simulink model "adaptive_feedforward"  (R2025b)
settings: Solver=FixedStepAuto  StartTime=0.0  StopTime=20  FixedStep=Ts  RelTol=1e-3
InitFcn:
  | design_adaptive_ff
values from neighbouring files (symbols this model uses):
  gamma = 1    [design_adaptive_ff.m]
  gamma_0 = 1    [design_adaptive_ff.m]
settings Model: Creator=10120  LastModifiedBy=10120

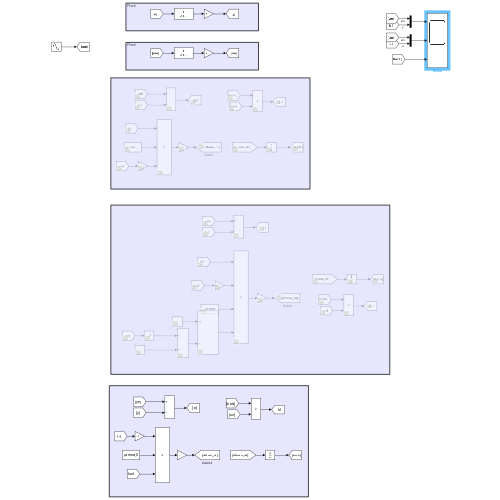
[thumbnail: Simulink's stored preview of the top-level diagram]
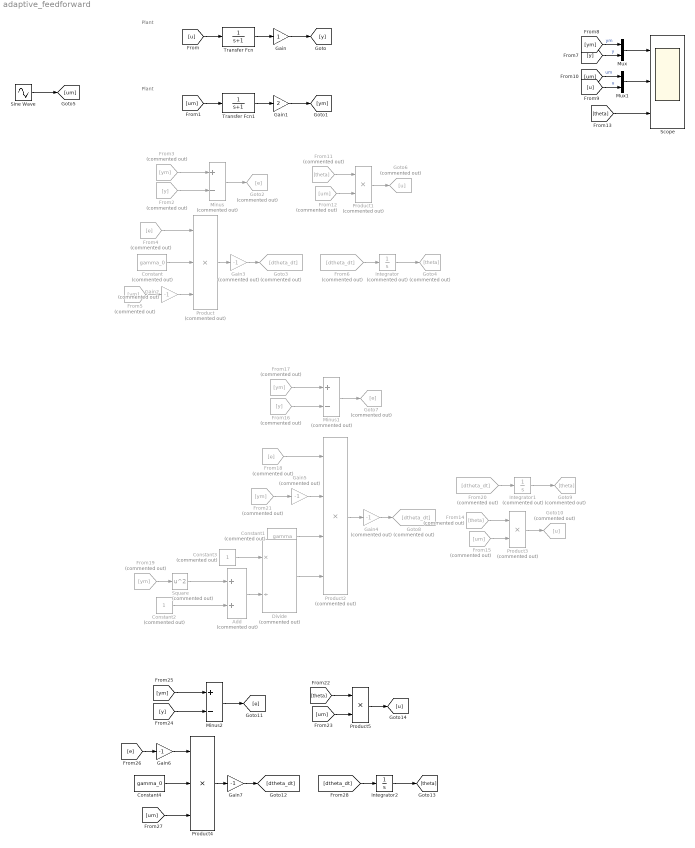
== system adaptive_feedforward ==
  note: Plant
  note: Plant
  Add : Sum  Commented=on
  Constant : Constant  Commented=on  Value=gamma_0
  Constant1 : Constant  Commented=on  Value=gamma
  Constant2 : Constant  Commented=on
  Constant3 : Constant  Commented=on
  Constant4 : Constant  Value=gamma_0
  Divide : Product  Commented=on  Inputs=*/
  From11 : From  Commented=on  GotoTag=theta
  From12 : From  Commented=on  GotoTag=um
  From14 : From  Commented=on  GotoTag=theta
  From15 : From  Commented=on  GotoTag=um
  From16 : From  Commented=on  GotoTag=y
  From{3,5,17,19,21} (5 alike) : From  Commented=on  GotoTag=ym
  From18 : From  Commented=on  GotoTag=e
  From2 : From  Commented=on  GotoTag=y
  From20 : From  Commented=on  GotoTag=dtheta_dt
  From4 : From  Commented=on  GotoTag=e
  From6 : From  Commented=on  GotoTag=dtheta_dt
  Gain : Gain
  Gain1 : Gain  Gain=2
  Gain{2..5} (4 alike) : Gain  Commented=on  Gain=-1
  Gain6 : Gain  Gain=-1
  Gain7 : Gain  Gain=-1
  Goto10 : Goto  Commented=on  GotoTag=u
  Goto2 : Goto  Commented=on  GotoTag=e
  Goto3 : Goto  Commented=on  GotoTag=dtheta_dt
  Goto4 : Goto  Commented=on  GotoTag=theta
  Goto6 : Goto  Commented=on  GotoTag=u
  Goto7 : Goto  Commented=on  GotoTag=e
  Goto8 : Goto  Commented=on  GotoTag=dtheta_dt
  Goto9 : Goto  Commented=on  GotoTag=theta
  Integrator : Integrator  Commented=on
  Integrator1 : Integrator  Commented=on
  Integrator2 : Integrator
  Minus : Sum  Commented=on  Inputs=+-
  Minus1 : Sum  Commented=on  Inputs=+-
  Minus2 : Sum  Inputs=+-
  Mux : Mux  Inputs=2
  Mux1 : Mux  Inputs=2
  Product : Product  Commented=on  Inputs=3
  Product1 : Product  Commented=on
  Product2 : Product  Commented=on  Inputs=4
  Product3 : Product  Commented=on
  Product4 : Product  Inputs=3
  Product5 : Product
  Scope : Scope  NumInputPorts=3
      settings: ActiveDisplayYMinimum=-1.7800302500498437  ActiveDisplayYMaximum=1.8782195801250892
  Sine Wave : Sin  SampleTime=0
  Square : Math  Commented=on  Operator=square
  Transfer Fcn : TransferFcn  Denominator=[1 1]
  Transfer Fcn1 : TransferFcn  Denominator=[1 1]
  wires:
  Transfer Fcn/1 -> Gain/1
  [u] -> Transfer Fcn/1
  Gain/1 -> [y]
  Gain1/1 -> [ym]
  [um] -> Transfer Fcn1/1
  Transfer Fcn1/1 -> Gain1/1
  From3/1 -> Minus/1
  From2/1 -> Minus/2
  Minus/1 -> Goto2/1
  From4/1 -> Product/1
  Constant/1 -> Product/2
  From5/1 -> Gain2/1
  Product/1 -> Gain3/1
  From6/1 -> Integrator/1
  Integrator/1 -> Goto4/1
  [ym] -> Mux/1  "ym"
  [y] -> Mux/2  "y"
  Mux/1 -> Scope/1
  [u] -> Mux1/2  "u"
  [um] -> Mux1/1  "um"
  Mux1/1 -> Scope/2
  Sine Wave/1 -> [um]
  From11/1 -> Product1/1
  From12/1 -> Product1/2
  Product1/1 -> Goto6/1
  [theta] -> Scope/3
  From14/1 -> Product3/1
  From15/1 -> Product3/2
  Product3/1 -> Goto10/1
  From16/1 -> Minus1/2
  From17/1 -> Minus1/1
  Product2/1 -> Gain4/1
  From20/1 -> Integrator1/1
  Constant1/1 -> Product2/3
  Integrator1/1 -> Goto9/1
  Minus1/1 -> Goto7/1
  From21/1 -> Gain5/1
  From19/1 -> Square/1
  Square/1 -> Add/1
  Constant2/1 -> Add/2
  Add/1 -> Divide/2
  Constant3/1 -> Divide/1
  Divide/1 -> Product2/4
  From18/1 -> Product2/1
  Gain2/1 -> Product/3
  Gain3/1 -> Goto3/1
  Gain4/1 -> Goto8/1
  Gain5/1 -> Product2/2
  [theta] -> Product5/1
  [um] -> Product5/2
  Product5/1 -> [u]
  [um] -> Product4/3
  Gain7/1 -> [dtheta_dt]
  [e] -> Gain6/1
  [y] -> Minus2/2
  [ym] -> Minus2/1
  Product4/1 -> Gain7/1
  [dtheta_dt] -> Integrator2/1
  Constant4/1 -> Product4/2
  Integrator2/1 -> [theta]
  Minus2/1 -> [e]
  Gain6/1 -> Product4/1
